simulink model "Levitatore_LQG_regulator"  (Simulink 7.5)
settings: Solver=ode45  StartTime=0.0  StopTime=3  FixedStep=Ts  MaxStep=1e-2  RelTol=1e-3
values from neighbouring files (symbols this model uses):
  d_w = 0.00005    (= 5e-05)    [TSC160127ProvaMatlab.m]
  d_y = 0.00001    (= 1e-05)    [TSC160127ProvaMatlab.m]
  dx0 = 0    [TSC160127ProvaMatlab.m]
  g = 9.81    [TSC160127ProvaMatlab.m]
  ie = sqrt((m*g*x0^2-k0)/km)    [TSC160127ProvaMatlab.m]
  k0 = 4    [TSC160127ProvaMatlab.m]
  km = 5    [TSC160127ProvaMatlab.m]
  kv = 1    [TSC160127ProvaMatlab.m]
  L = -LKalman    [TSC160127ProvaMatlab.m]
  m = 5    [TSC160127ProvaMatlab.m]
  v0 = 2    [TSC160127ProvaMatlab.m]
  x0 = 0.5 + 0.03    (= 0.53)    [TSC160127ProvaMatlab.m]
  ye = kv * x0 + v0    (= 2.5)    [TSC160127ProvaMatlab.m]
undefined symbols (not defined in the file or in its folder): A, B, C, K
settings Model: Creator=lbiagiotti  LastModifiedBy=Biagio
settings DebuggingCC: SaveWithParameterizedLinksMsg=none  StrictBusMsg=Warning
settings HardwareCC: TargetHWDeviceType=32-bit Generic
settings GRTTargetCC: TargetFcnLib=ansi_tfl_tmw.mat

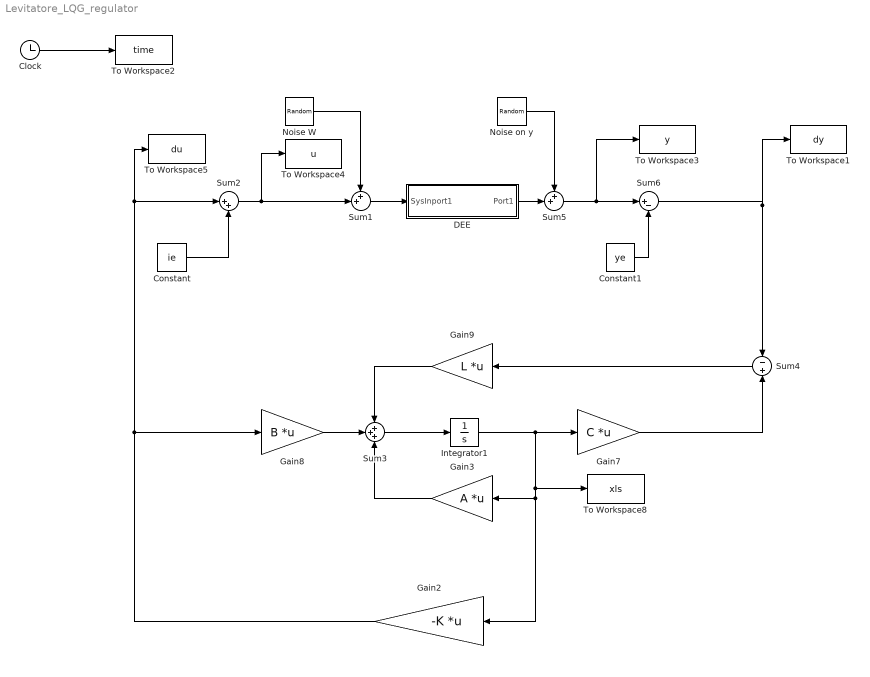
== system Levitatore_LQG_regulator ==
  Clock : Clock
      settings: Decimation=10
  Constant : Constant  Value=ie  OutDataType=sfix(16)  OutScaling=2^0
  Constant1 : Constant  Value=ye  OutDataType=sfix(16)  OutScaling=2^0
  DEE : Subsystem
      settings: OpenFcn=diffeqed
      mask Type: Differential Equation Editor (DEE)
      mask Display: disp('Levitatore')
  Gain2 : Gain  Gain=-K  Multiplication=Matrix(K*u)  ParameterDataType=sfix(16)  ParameterScaling=2^0  OutDataType=sfix(16)  OutScaling=2^0
  Gain3 : Gain  Gain=A  Multiplication=Matrix(K*u)  ParameterDataType=sfix(16)  ParameterScaling=2^0  OutDataType=sfix(16)  OutScaling=2^0
  Gain7 : Gain  Gain=C  Multiplication=Matrix(K*u)  ParameterDataType=sfix(16)  ParameterScaling=2^0  OutDataType=sfix(16)  OutScaling=2^0
  Gain8 : Gain  Gain=B  Multiplication=Matrix(K*u)  ParameterDataType=sfix(16)  ParameterScaling=2^0  OutDataType=sfix(16)  OutScaling=2^0
  Gain9 : Gain  Gain=L  Multiplication=Matrix(K*u)  ParameterDataType=sfix(16)  ParameterScaling=2^0  OutDataType=sfix(16)  OutScaling=2^0
  Integrator1 : Integrator  InitialCondition=[0 0]'
  Noise W : RandomNumber  Variance=d_w  SampleTime=0
  Noise on y : RandomNumber  Variance=d_y  SampleTime=0
  Sum1 : Sum  Inputs=++|  OutDataType=fixdt(1, 16)  OutScaling=2^0
  Sum2 : Sum  Inputs=|++  OutDataType=sfix(16)  OutScaling=2^0
  Sum3 : Sum  Inputs=+++  OutDataType=sfix(16)  OutScaling=2^0
  Sum4 : Sum  Inputs=-+  OutDataType=sfix(16)  OutScaling=2^0
  Sum5 : Sum  Inputs=++|  OutDataType=fixdt(1, 16)  OutScaling=2^0
  Sum6 : Sum  Inputs=|+-  OutDataType=sfix(16)  OutScaling=2^0
  To Workspace1 : ToWorkspace  VariableName=dy  SampleTime=-1  SaveFormat=Array
  To Workspace2 : ToWorkspace  VariableName=time  SampleTime=-1  SaveFormat=Array
  To Workspace3 : ToWorkspace  VariableName=y  SampleTime=-1  SaveFormat=Array
  To Workspace4 : ToWorkspace  VariableName=u  SampleTime=-1  SaveFormat=Array
  To Workspace5 : ToWorkspace  VariableName=du  SampleTime=-1  SaveFormat=Array
  To Workspace8 : ToWorkspace  VariableName=xls  SampleTime=-1  SaveFormat=Array
  wires:
  Clock/1 -> To Workspace2/1
  Gain2/1 -> Gain8/1, To Workspace5/1, Sum2/1
  Sum3/1 -> Integrator1/1
  Integrator1/1 -> Gain7/1, To Workspace8/1, Gain3/1, Gain2/1
  Gain7/1 -> Sum4/2
  Gain9/1 -> Sum3/1
  Gain8/1 -> Sum3/2
  Gain3/1 -> Sum3/3
  Sum4/1 -> Gain9/1
  Noise W/1 -> Sum1/1
  Sum1/1 -> DEE/1(SysInport1)
  Noise on y/1 -> Sum5/1
  DEE/1(Port1) -> Sum5/2
  Constant/1 -> Sum2/2
  Sum2/1 -> Sum1/2, To Workspace4/1
  Sum5/1 -> Sum6/1, To Workspace3/1
  Constant1/1 -> Sum6/2
  Sum6/1 -> Sum4/1, To Workspace1/1

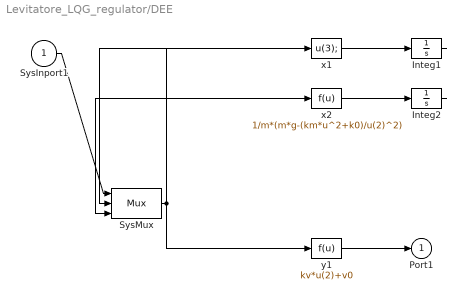
== system Levitatore_LQG_regulator/DEE ==
  SysInport1 : Inport
  Integ1 : Integrator  InitialCondition=x0
  Integ2 : Integrator  InitialCondition=dx0
  SysMux : Mux  Inputs=3
  x1 : Fcn  Expr=u(3);
  x2 : Fcn  Expr=1/m*(m*g-(km*u^2+k0)/u(2)^2)
  y1 : Fcn  Expr=kv*u(2)+v0
  Port1 : Outport
  wires:
  SysInport1/1 -> SysMux/1
  SysMux/1 -> x1/1, x2/1, y1/1
  x1/1 -> Integ1/1
  Integ1/1 -> SysMux/2
  x2/1 -> Integ2/1
  Integ2/1 -> SysMux/3
  y1/1 -> Port1/1
